simulink subsystem "Gearbox"  (R2023a)
settings: Solver=VariableStepAuto  StartTime=0.0  StopTime=10.0  RelTol=1e-3
model mask{i_gear=0, J_gear=0, vis_friction_coef_gear=0}
  mask prompts: i_gear "gear ratio"; J_gear "Inertion of gearbox"; vis_friction_coef_gear "Coef of viscous friction"
settings Model: Creator=ПК  LastModifiedBy=ПК

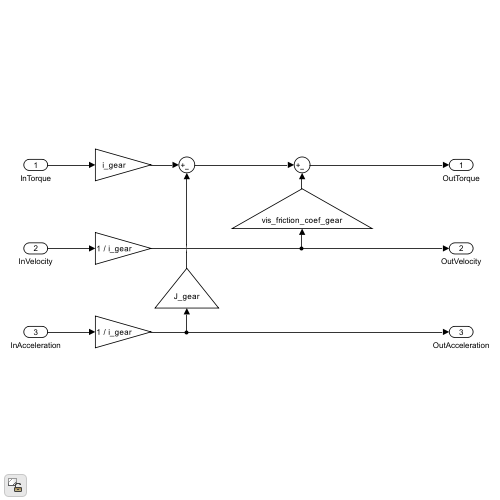
[thumbnail: Simulink's stored preview of the top-level diagram]
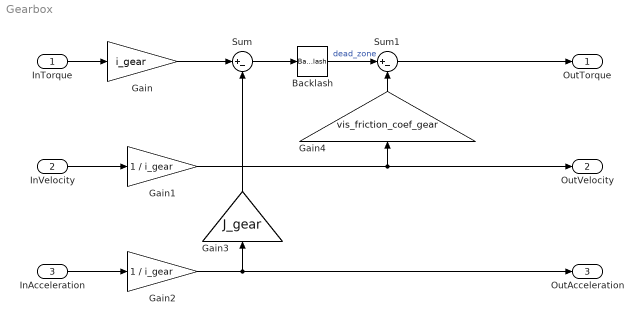
== system Gearbox ==
  InTorque : Inport
  InVelocity : Inport  Port=2
  InAcceleration : Inport  Port=3
  Backlash : Backlash  BacklashWidth=0.5
  Gain : Gain  Gain=i_gear
  Gain1 : Gain  Gain=1 / i_gear
  Gain2 : Gain  Gain=1 / i_gear
  Gain3 : Gain  Gain=J_gear
  Gain4 : Gain  Gain=vis_friction_coef_gear
  Sum : Sum  Inputs=|+-
  Sum1 : Sum  Inputs=|+-
  OutTorque : Outport
  OutVelocity : Outport  Port=2
  OutAcceleration : Outport  Port=3
  wires:
  InTorque/1 -> Gain/1
  InVelocity/1 -> Gain1/1
  InAcceleration/1 -> Gain2/1
  Gain2/1 -> OutAcceleration/1, Gain3/1
  Gain1/1 -> OutVelocity/1, Gain4/1
  Gain/1 -> Sum/1
  Sum1/1 -> OutTorque/1
  Gain3/1 -> Sum/2
  Gain4/1 -> Sum1/2
  Sum/1 -> Backlash/1
  Backlash/1 -> Sum1/1  "dead_zone"
